simulink model "Projectilev1"  (R2022b)
settings: Solver=VariableStepAuto  StartTime=0.0  StopTime=12  RelTol=1e-3
libraries: vrlib x1
settings Model: Creator=ASUS  LastModifiedBy=ASUS

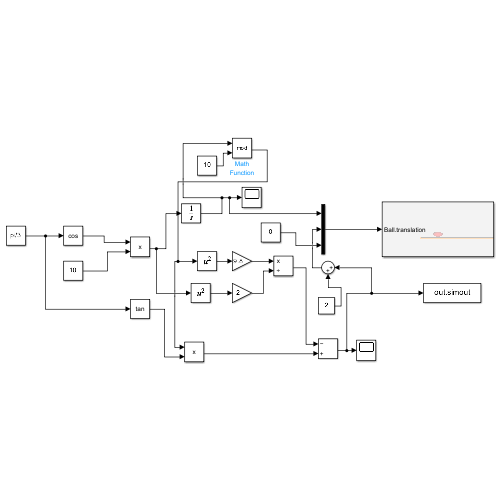
[thumbnail: Simulink's stored preview of the top-level diagram]
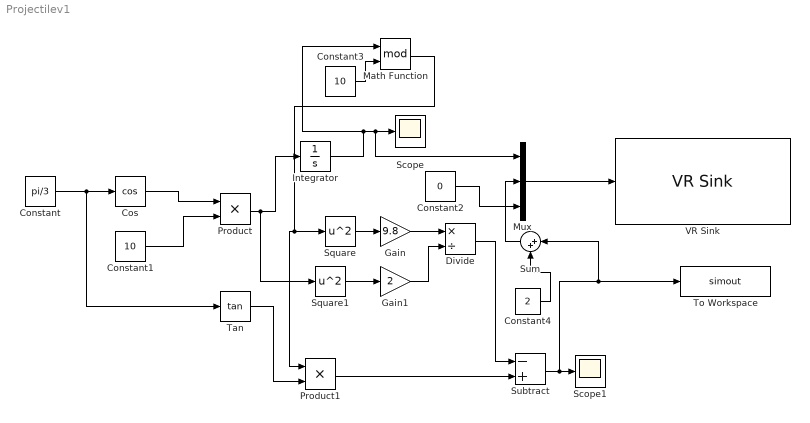
== system Projectilev1 ==
  Constant : Constant  Value=pi/3
  Constant1 : Constant  Value=10
  Constant2 : Constant  Value=0
  Constant3 : Constant  Value=10
  Constant4 : Constant  Value=2
  Cos : Trigonometry  Operator=cos
  Divide : Product  Inputs=*/
  Gain : Gain  Gain=9.8
  Gain1 : Gain  Gain=2
  Integrator : Integrator
  Math Function : Math  Operator=mod
  Mux : Mux  Inputs=3
  Product : Product
  Product1 : Product
  Scope : Scope
  Scope1 : Scope
  Square : Math  Operator=square
  Square1 : Math  Operator=square
  Subtract : Sum  Inputs=-+
  Sum : Sum  Inputs=|++
  Tan : Trigonometry  Operator=tan
  To Workspace : ToWorkspace  VariableName=simout  SaveFormat=Timeseries  SampleTime=-1
  VR Sink : vrlib/VR Sink  InstantiateOnLoad=on  SampleTime=0.1  ViewEnable=on  RemoteChange=off  RemoteView=off  FieldsWritten=Ball.translation.3.1.1.double  WorldFileName=Ball.x3d  WorldDescription=VR Bouncing Ball  AutoView=off  VideoDimensions=[]  AllowVariableSize=off  FigureProperties="{'Position', 'Name', 'Viewpoint', 'CameraBound', 'CameraDirection', 'CameraPosition', 'CameraUpVector', 'ZoomFactor', 'Antialiasing', 'Headlight', 'Lighting', 'NavPanel', 'Sound', 'StatusBar', 'Stereo3D', 'Stereo3DCameraOffset', 'Stereo3DHIT', 'ToolBar', 'Textures', 'Transparency', 'Triad', 'Wireframe', 'NavZones', 'NavMode', 'NavSpeed', 'CaptureFileFormat', 'CaptureFileName', 'Record2DCompressMethod', 'Record2DCompressQuality', 'Record2D', 'Record2DFileName', 'Record2DFPS'; [7.6980000000000007e+02   8.1399999999999977e+01   7.6640000000000020e+02   7.3080000000000007e+02], 'VR Bouncing Ball', 'Ball', 'on', [5.6464247339503559e-01   0.0000000000000000e+00  -8.2533561490967877e-01], [-4.2912827978022669e+01   0.0000000000000000e+00   6.2725506733135504e+01], [0.0000000000000000e+00   1.0000000000000000e+00   0.0000000000000000e+00], [1.0000000000000000e+00], 'on', 'on', 'on', 'halfbar', 'on', 'on', 'off', [1.0000000149011612e-01], [0.0000000000000000e+00], 'on', 'on', 'on', 'none', 'off', 'off', 'examine', 'normal', 'tif', '%f_anim_%n.tif', 'auto', [7.5000000000000000e+01], 'off', '%f_anim_%n.avi', 'auto'}"
  wires:
  Constant/1 -> Tan/1, Cos/1
  Cos/1 -> Product/1
  Product/1 -> Square1/1, Integrator/1
  Constant1/1 -> Product/2
  Tan/1 -> Product1/2
  Product1/1 -> Subtract/2
  Square/1 -> Gain/1
  Gain/1 -> Divide/1
  Square1/1 -> Gain1/1
  Gain1/1 -> Divide/2
  Divide/1 -> Subtract/1
  Integrator/1 -> Math Function/1, Mux/1, Scope/1
  Constant2/1 -> Mux/3
  Mux/1 -> VR Sink/1
  Constant3/1 -> Math Function/2
  Math Function/1 -> Square/1, Product1/1
  Subtract/1 -> Sum/1, To Workspace/1, Scope1/1
  Constant4/1 -> Sum/2
  Sum/1 -> Mux/2
